simulink model "PubIfDecisionTOS_MDL"  (R2020b)
settings: configuration reference "DspaceConfig" (kept outside this file)
PostLoadFcn:
  | if any(exist('dsrtsu_mdlpostloadfcn', 'file') ~= 0), dsrtsu_mdlpostloadfcn('Execute', bdroot); end
InitFcn:
  | , if any(exist('dsmpb_private', 'file') ~= 0), dsmpb_private('dsmpb_mdlclblib', 'Init', bdroot); end,
undefined symbols (not defined in the file or in its folder): C_TOS_ACCEgoRAxletoFbumplength_m, C_TOS_ACCTargetFront_Flag, C_TOS_AEBJAPedObjDxThre_Val, C_TOS_AEBJAPedObjDyThre_Val, C_TOS_AEBJATargetSize_Val, C_TOS_AEBJAVehObjDxThre_Val, C_TOS_AEBJAVehObjDyThre_Val, C_TOS_AEBJuncPedTargetSize_Val, C_TOS_AEBLatObjDxThre_Val, C_TOS_AEBLatPedDyThre_Val, C_TOS_AEBLatTargetSize_Val, C_TOS_AEBLongTargetInEgoFront_Flag, C_TOS_axAbsGround_Parameter, C_TOS_CameraConfirmedFlag, C_TOS_CNsubjWidth, C_TOS_CurrentLaneCoreMinWidth_Val, C_TOS_CutInProb_Val_Zero, C_TOS_CutOutProb_Val_Zero, C_TOS_D2R_Val, C_TOS_DefaultValueObjectToCenterLine_dy, C_TOS_EgoCarWidth_Val, C_TOS_EgoDxRefPoint_m, C_TOS_EgoRAxletoFbumplength_m, C_TOS_HalfWidthVehicle_Con, C_TOS_HWA_CurrentLaneFlag, C_TOS_HWA_LeftLaneFlag, C_TOS_HWA_MovingDir_Vaild, C_TOS_HWA_MovState_Vaild, C_TOS_HWA_RightLaneFlag, C_TOS_LaneLineCourseErrorFront, C_TOS_LaneLineCourseErrorRear, C_TOS_MotorbikeDefaultWidth_m, C_TOS_NumberOfEffectiveTargets, C_TOS_Obj_Age_Val, C_TOS_Objdx_Constraint_Val, C_TOS_ObjectDefaultWidth_m, C_TOS_ObjInCurrentLane_Val, C_TOS_ObjInCurrentLaneValid, C_TOS_ObjInLeftLaneValid, C_TOS_ObjInRightLaneValid, C_TOS_ObjNotInCurrentLane_Val, C_TOS_ObjNotREElementType, C_TOS_ObjPredictDis_dy_ConstantVal_Zeros, C_TOS_ObjToCenterLine_ConstantVal_Zeros, C_TOS_OFMObjIDInvilad_Val, C_TOS_PIL_LatDisCons_Val_zero, C_TOS_PIL_ObjectCutInFlag_b, C_TOS_PIL_ObjectCutOutFlag_b, C_TOS_PIL_ObjLaneProb_al_Val, C_TOS_PP_ObjFusType_FC_Confirm_b, C_TOS_PP_ObjFusType_FC_FR_Confirm_b, C_TOS_PP_ObjFusType_FR_Confirm_b, C_TOS_RE_80BoolDefault_Val, C_TOS_RE_80Single181Default_Val, C_TOS_RE_80Single255Default_Val, C_TOS_RE_80Uint8Default_Val, C_TOS_RE_D2R, C_TOS_RE_D_180_Val, C_TOS_RE_InvalidObjectID_Val, C_TOS_RE_InvalidTargetChainDir_Val ... (+142)
libraries: simulink x1650, TOS_LIB x361, canfdmsglib x14
(part 22 of 69)

== system PubIfDecisionTOS_MDL/TOS_20201112/TOS_2012080320/TOS/LC_LCKie_ELK/TOS_HWA/CurrentLane/HWA_Object_PreConfirm ==
  PP_ObjFusType_FC_FR_Confirm : Inport
  PP_ObjFusType_FR_Confirm : Inport  Port=2
  PP_ObjFusType_FC_Confirm : Inport  Port=3
  Object_ID : Inport  Port=4
  Obj_MovingState : Inport  Port=5
  Obj_Dx : Inport  Port=6
  Object_ObstacleProb : Inport  Port=7
  Object_DY : Inport  Port=8
  Object_Type : Inport  Port=9
  TOS_TLJ_SameLaneConfirm_Flag : Inport  Port=10
  LM_LR_Line04_fCamValid : Inport  Port=11
  LM_LR_Line05_fCamValid : Inport  Port=12
  LM_LR_Line06_fCamValid : Inport  Port=13
  PIL_OverlapRatio : Inport  Port=14
  LM_LR_Line04_dDisStart : Inport  Port=15
  LM_LR_Line04_dDisEnd : Inport  Port=16
  LM_LR_Line05_dDisStart : Inport  Port=17
  LM_LR_Line05_dDisEnd : Inport  Port=18
  LM_LR_Line06_dDisStart : Inport  Port=19
  LM_LR_Line06_dDisEnd : Inport  Port=20
  TOS_HWA_CurrentFront_Target_2_ID_K1 : Inport  Port=21
  TOS_HWA_CurrentFront_Target_2_Dx_K1 : Inport  Port=22
  Bus Creator : BusCreator  Inputs=10
  Constant : Constant  Value=10  OutDataTypeStr=uint8
  Delay : Delay  InitialCondition=0
  Selector1 : Selector  InputPortWidth=11  IndexOptions=Index vector (port)  Indices=[1 3]  OutputSizes=1
  Selector2 : Selector  InputPortWidth=11  IndexOptions=Index vector (port)  Indices=[1 3]  OutputSizes=1
  TOS_HWA_CurrentLaneFront_TargPreConfirm : Subsystem
  Unit Delay : UnitDelay  SampleTime=-1  HasFrameUpgradeWarning=on
  Unit Delay1 : UnitDelay  InitialCondition=255  SampleTime=-1  HasFrameUpgradeWarning=on
  Unit Delay2 : UnitDelay  SampleTime=-1  HasFrameUpgradeWarning=on
  TOS_HWA_CLF_TargetPreConfirm : Outport
  wires:
  PP_ObjFusType_FR_Confirm/1 -> TOS_HWA_CurrentLaneFront_TargPreConfirm/2(PP_ObjFusType_FR_Confirm)
  PP_ObjFusType_FC_FR_Confirm/1 -> TOS_HWA_CurrentLaneFront_TargPreConfirm/1(PP_ObjFusType_FC_FR_Confirm)
  PP_ObjFusType_FC_Confirm/1 -> TOS_HWA_CurrentLaneFront_TargPreConfirm/3(PP_ObjFusType_FC_Confirm)
  Object_ID/1 -> TOS_HWA_CurrentLaneFront_TargPreConfirm/4(Object_ID)
  TOS_HWA_CurrentFront_Target_2_Dx_K1/1 -> Selector2/1
  TOS_HWA_CurrentFront_Target_2_ID_K1/1 -> Selector1/1
  Object_DY/1 -> TOS_HWA_CurrentLaneFront_TargPreConfirm/8(Object_DY)
  Object_ObstacleProb/1 -> TOS_HWA_CurrentLaneFront_TargPreConfirm/7(Object_ObstacleProb)
  Obj_Dx/1 -> TOS_HWA_CurrentLaneFront_TargPreConfirm/6(Obj_Dx)
  Obj_MovingState/1 -> TOS_HWA_CurrentLaneFront_TargPreConfirm/5(Obj_MovingState)
  Object_Type/1 -> TOS_HWA_CurrentLaneFront_TargPreConfirm/9(Object_ObjType)
  Bus Creator/1 -> TOS_HWA_CLF_TargetPreConfirm/1  "TOS_HWA_CLF_TargetPre_ObserVale"
  PIL_OverlapRatio/1 -> Delay/1, Unit Delay2/1, TOS_HWA_CurrentLaneFront_TargPreConfirm/16(PIL_OverlapRatio)
  TOS_TLJ_SameLaneConfirm_Flag/1 -> TOS_HWA_CurrentLaneFront_TargPreConfirm/10(TOS_TLJ_SameLaneConfirm_Flag)
  TOS_HWA_CurrentLaneFront_TargPreConfirm/1(TOS_HWA_TargetPre_Filt_Flag) -> Bus Creator/1  "TOS_HWA_CLF_TargetPre_Filt_Flag"
  TOS_HWA_CurrentLaneFront_TargPreConfirm/2(TOS_HWA_TargetPre_1_ConditionFlag_ObserVale) -> Bus Creator/2  "TOS_HWA_CLF_TargetPre_1_ConditionFlag_ObserVale"
  TOS_HWA_CurrentLaneFront_TargPreConfirm/3(TOS_HWA_TargetPre_FusionTypeFlag_ObserVale) -> Bus Creator/3  "TOS_HWA_CLF_TargetPre_FusionTypeFlag_ObserVale"
  TOS_HWA_CurrentLaneFront_TargPreConfirm/4(TOS_HWA_TargetPre_PassedbyTarget_Flag_ObserVale) -> Bus Creator/4  "TOS_HWA_CLF_TargetPre_PassedbyTarget_Flag_ObserVale"
  TOS_HWA_CurrentLaneFront_TargPreConfirm/5(TOS_HWA_TargetPre_FenceFlag_ObserVale) -> Bus Creator/5  "TOS_HWA_CLF_TargetPre_FenceFlag_ObserVale"
  TOS_HWA_CurrentLaneFront_TargPreConfirm/6(TOS_HWA_TargetPre_ObjType_ObserVale) -> Bus Creator/6  "TOS_HWA_CLF_TargetPre_ObjType_ObserVale"
  TOS_HWA_CurrentLaneFront_TargPreConfirm/7(TOS_HWA_TargetPre_OverlapThre_Val_ObserVale) -> Bus Creator/7  "TOS_HWA_CLF_TargetPre_OverlapThre_Val_ObserVale"
  TOS_HWA_CurrentLaneFront_TargPreConfirm/8(TOS_HWA_TargetPre_SameLane_Flag) -> Bus Creator/8  "TOS_HWA_CLF_TargetPre_SameLane_Flag"
  TOS_HWA_CurrentLaneFront_TargPreConfirm/9(TOS_HWA_TargetPre_2_OverlapThre_ObserVale) -> Bus Creator/9  "TOS_HWA_CLF_TargetPre_2_OverlapThre_ObserVale"
  TOS_HWA_CurrentLaneFront_TargPreConfirm/10(TOS_HWA_TargetPre_3_SameLane_Flag_ObserVale) -> Bus Creator/10  "TOS_HWA_CLF_TargetPre_3_SameLane_Flag_ObserVale"
  Unit Delay/1 -> TOS_HWA_CurrentLaneFront_TargPreConfirm/14(TOS_HWA_CurrentFront_Target_2_ID_K1)
  Unit Delay1/1 -> TOS_HWA_CurrentLaneFront_TargPreConfirm/15(TOS_HWA_Dx_K1)
  Unit Delay2/1 -> TOS_HWA_CurrentLaneFront_TargPreConfirm/17(PIL_OverlapRatio_K1)
  Delay/1 -> TOS_HWA_CurrentLaneFront_TargPreConfirm/18(PIL_OverlapRatio_K2)
  LM_LR_Line04_fCamValid/1 -> TOS_HWA_CurrentLaneFront_TargPreConfirm/11(LM_LR_Line04_fCamValid)
  LM_LR_Line05_fCamValid/1 -> TOS_HWA_CurrentLaneFront_TargPreConfirm/12(LM_LR_Line05_fCamValid)
  LM_LR_Line06_fCamValid/1 -> TOS_HWA_CurrentLaneFront_TargPreConfirm/13(LM_LR_Line06_fCamValid)
  LM_LR_Line06_dDisEnd/1 -> TOS_HWA_CurrentLaneFront_TargPreConfirm/24(LM_LR_Line06_dDisEnd)
  LM_LR_Line04_dDisStart/1 -> TOS_HWA_CurrentLaneFront_TargPreConfirm/19(LM_LR_Line04_dDisStart)
  LM_LR_Line04_dDisEnd/1 -> TOS_HWA_CurrentLaneFront_TargPreConfirm/20(LM_LR_Line04_dDisEnd)
  LM_LR_Line05_dDisStart/1 -> TOS_HWA_CurrentLaneFront_TargPreConfirm/21(LM_LR_Line05_dDisStart)
  LM_LR_Line05_dDisEnd/1 -> TOS_HWA_CurrentLaneFront_TargPreConfirm/22(LM_LR_Line05_dDisEnd)
  LM_LR_Line06_dDisStart/1 -> TOS_HWA_CurrentLaneFront_TargPreConfirm/23(LM_LR_Line06_dDisStart)
  Selector1/1 -> Unit Delay/1
  Selector2/1 -> Unit Delay1/1
  Constant/1 -> Selector1/2, Selector2/2

== system PubIfDecisionTOS_MDL/TOS_20201112/TOS_2012080320/TOS/LC_LCKie_ELK/TOS_HWA/LeftLane/HWA_Object_PreConfirm ==
  PP_ObjFusType_FC_FR_Confirm : Inport
  PP_ObjFusType_FR_Confirm : Inport  Port=2
  PP_ObjFusType_FC_Confirm : Inport  Port=3
  Object_ID : Inport  Port=4
  Obj_MovingState : Inport  Port=5
  Obj_Dx : Inport  Port=6
  Object_ObstacleProb : Inport  Port=7
  Object_DY : Inport  Port=8
  Object_Type : Inport  Port=9
  Bus Creator : BusCreator  Inputs=5
  HWA_Object_PreConfirm : Subsystem
  TOS_HWA_LLF_TargetPreConfirm : Outport
  wires:
  PP_ObjFusType_FR_Confirm/1 -> HWA_Object_PreConfirm/2(PP_ObjFusType_FR_Confirm)
  PP_ObjFusType_FC_FR_Confirm/1 -> HWA_Object_PreConfirm/1(PP_ObjFusType_FC_FR_Confirm)
  PP_ObjFusType_FC_Confirm/1 -> HWA_Object_PreConfirm/3(PP_ObjFusType_FC_Confirm)
  Object_ID/1 -> HWA_Object_PreConfirm/4(Object_ID)
  Object_DY/1 -> HWA_Object_PreConfirm/8(Object_DY)
  Object_ObstacleProb/1 -> HWA_Object_PreConfirm/7(Object_ObstacleProb)
  Obj_Dx/1 -> HWA_Object_PreConfirm/6(Obj_Dx)
  Obj_MovingState/1 -> HWA_Object_PreConfirm/5(Obj_MovingState)
  Object_Type/1 -> HWA_Object_PreConfirm/9(Object_ObjType)
  Bus Creator/1 -> TOS_HWA_LLF_TargetPreConfirm/1  "TOS_HWA_LLF_TargetPreConfirm"
  HWA_Object_PreConfirm/1(TOS_HWA_TargetPre_Confirm_Filt_Flag) -> Bus Creator/1  "TOS_HWA_LLF_TargetPre_Confirm_Filt_Flag"
  HWA_Object_PreConfirm/2(TOS_HWA_TargetPre_FusionTypeFlag_ObserVale) -> Bus Creator/2  "TOS_HWA_LLF_TargetPre_FusionTypeFlag_ObserVale"
  HWA_Object_PreConfirm/3(TOS_HWA_TargetPre_PassedbyTarget_ObserVale) -> Bus Creator/3  "TOS_HWA_LLF_TargetPre_PassedbyTarget_ObserVale"
  HWA_Object_PreConfirm/4(TOS_HWA_TargetPre_ObjType_ObserVale) -> Bus Creator/4  "TOS_HWA_LLF_TargetPre_ObjType_ObserVale"
  HWA_Object_PreConfirm/5(TOS_HWA_DyConfirm_ObserVale) -> Bus Creator/5  "TOS_HWA_LLF_DyConfirm_ObserVale"

== system PubIfDecisionTOS_MDL/TOS_20201112/TOS_2012080320/TOS/LC_LCKie_ELK/TOS_HWA/LeftLane/TOS_HWA_LeftLane ==
  TOSAAt_OFM_TIL_VIE : Inport
  HWA_LeftLane_ObjIndex : Inport  Port=2
  Bus Creator : BusCreator  Inputs=2
  Bus Creator1 : BusCreator  Inputs=5
  Bus Creator2 : BusCreator  Inputs=3
  Bus Selector : BusSelector  OutputSignals=TOS_AddAttributes.PP_ObjMovingDirSignalProcessing,OFM_SignalVerification.Object_VX,OFM_SignalVerification.Object_VY,OFM_SignalVerification.Object_Type,OFM_SignalVerification.Object_MovingState,TLJ_TargetInLaneValidityJudg.TOS_TLJ_LeftLaneConfirm_Flag,OFM_SignalVerification.Object_DX,OFM_SignalVerification.Object_DY,OFM_SignalVerification.Object_Fus_Type,OFM_SignalVerification.Object_HeadingAngle,TOS_AddAttributes.PP_ObjFusType_FC_FR_Confirm,TOS_AddAttributes.PP_ObjFusType_FR_Confirm,TOS_AddAttributes.PP_ObjFusType_FC_Confirm,VIE_SignalVerification.vxvRefMs
  Selector2 : Selector  InputPortWidth=4  IndexOptions=Index vector (dialog)  Indices=[1]  OutputSizes=1
  Selector3 : Selector  InputPortWidth=4  IndexOptions=Index vector (dialog)  Indices=[2]  OutputSizes=1
  Selector6 : Selector  InputPortWidth=4  IndexOptions=Index vector (dialog)  Indices=[3]  OutputSizes=1
  Selector7 : Selector  InputPortWidth=4  IndexOptions=Index vector (dialog)  Indices=[4]  OutputSizes=1
  TOS_HWA_LeftLane : Subsystem
  Terminator4 : Terminator
  HWA_LeftFront_Target_1 : Outport
  HWA_LeftFront_Target_2 : Outport  Port=2
  HWA_LeftRear_Target_3 : Outport  Port=3
  HWA_LeftRear_Target_4 : Outport  Port=4
  TargetInLeftLane_b : Outport  Port=5
  wires:
  TOS_HWA_LeftLane/11(TOS_HWA_LeftRear_DyConfirm_ObserVale) -> Bus Creator1/5  "TOS_HWA_LeftRear_DyConfirm_ObserVale"
  TOS_HWA_LeftLane/10(TOS_HWA_LeftRear_TargetMovingDir_ObserVale) -> Bus Creator1/4  "TOS_HWA_LeftRear_TargetMovingDir_ObserVale"
  TOS_HWA_LeftLane/9(TOS_HWA_InLeftLane_Rear_Flag_ObserVale) -> Bus Creator1/3  "TOS_HWA_InLeftLane_Rear_Flag_ObserVale"
  TOS_HWA_LeftLane/8(TOS_HWA_LeftRear_FusionType_ObserVale) -> Bus Creator1/2  "TOS_HWA_LeftRear_FusionType_ObserVale"
  TOS_HWA_LeftLane/7(TOS_HWA_LeftRear_MovState_ObserVale) -> Bus Creator1/1  "TOS_HWA_LeftRear_MovState_ObserVale"
  TOS_HWA_LeftLane/6(TOS_HWA_LeftFront_TargMovDir_ObserVale) -> Bus Creator2/3  "TOS_HWA_LeftFront_TargMovDir_ObserVale"
  TOS_HWA_LeftLane/5(TOS_HWA_InLeftLane_Front_Flag_ObserVale) -> Bus Creator2/2  "TOS_HWA_InLeftLane_Front_Flag_ObserVale"
  TOS_HWA_LeftLane/4(TOS_HWA_LeftFront_FusType_ObserVale) -> Bus Creator2/1  "TOS_HWA_LeftFront_FusType_ObserVale"
  Bus Selector/8 -> TOS_HWA_LeftLane/9(Object_DY)  "<Object_DY>"
  Bus Creator2/1 -> Bus Creator/1  "HWA_LeftLane_Front_ObserVale"
  Bus Creator1/1 -> Bus Creator/2  "HWA_LeftLane_Rear_ObserVale"
  TOS_HWA_LeftLane/3(TOS_HWA_LeftRear_TargConfirm_b) -> Selector7/1, Selector6/1
  Bus Selector/7 -> TOS_HWA_LeftLane/8(Object_DX)  "<Object_DX>"
  Bus Creator/1 -> Terminator4/1  "TOS_HWA_LeftLane_ObserVale"
  Bus Selector/14 -> TOS_HWA_LeftLane/15(VIE_EgoVelocity)  "<vxvRefMs>"
  Bus Selector/13 -> TOS_HWA_LeftLane/14(PP_ObjFusType_FC_Confirm)  "<PP_ObjFusType_FC_Confirm>"
  Bus Selector/12 -> TOS_HWA_LeftLane/13(PP_ObjFusType_FR_Confirm)  "<PP_ObjFusType_FR_Confirm>"
  Bus Selector/11 -> TOS_HWA_LeftLane/12(PP_ObjFusType_FC_FR_Confirm)  "<PP_ObjFusType_FC_FR_Confirm>"
  Selector2/1 -> HWA_LeftFront_Target_1/1
  Selector3/1 -> HWA_LeftFront_Target_2/1
  TOS_HWA_LeftLane/2(TOS_HWA_LeftFront_TargConfirm_b) -> Selector3/1, Selector2/1
  Selector7/1 -> HWA_LeftRear_Target_4/1
  Selector6/1 -> HWA_LeftRear_Target_3/1
  HWA_LeftLane_ObjIndex/1 -> TOS_HWA_LeftLane/1(HLeftLane_ObjIndex)
  TOSAAt_OFM_TIL_VIE/1 -> Bus Selector/1
  Bus Selector/1 -> TOS_HWA_LeftLane/2(PP_ObjMovingDirSignalProcessing)  "<PP_ObjMovingDirSignalProcessing>"
  Bus Selector/2 -> TOS_HWA_LeftLane/3(Object_VX)  "<Object_VX>"
  Bus Selector/3 -> TOS_HWA_LeftLane/4(Object_VY)  "<Object_VY>"
  Bus Selector/4 -> TOS_HWA_LeftLane/5(Object_Type)  "<Object_Type>"
  Bus Selector/5 -> TOS_HWA_LeftLane/6(Object_MovingState)  "<Object_MovingState>"
  Bus Selector/6 -> TOS_HWA_LeftLane/7(TOS_TLJ_LeftLaneConfirm_Flag)  "<TOS_TLJ_LeftLaneConfirm_Flag>"
  Bus Selector/9 -> TOS_HWA_LeftLane/10(Object_Fus_Type)  "<Object_Fus_Type>"
  TOS_HWA_LeftLane/1(TOS_HWA_TargetInLeftLane_b) -> TargetInLeftLane_b/1
  Bus Selector/10 -> TOS_HWA_LeftLane/11(Object_HeadingAngle)  "<Object_HeadingAngle>"

== system PubIfDecisionTOS_MDL/TOS_20201112/TOS_2012080320/TOS/LC_LCKie_ELK/TOS_HWA/RightLane/HWA_Object_PreConfirm ==
  PP_ObjFusType_FC_FR_Confirm : Inport
  PP_ObjFusType_FR_Confirm : Inport  Port=2
  PP_ObjFusType_FC_Confirm : Inport  Port=3
  Object_ID : Inport  Port=4
  Obj_MovingState : Inport  Port=5
  Obj_Dx : Inport  Port=6
  Object_ObstacleProb : Inport  Port=7
  Object_DY : Inport  Port=8
  Object_Type : Inport  Port=9
  Bus Creator : BusCreator  Inputs=5
  HWA_Object_PreConfirm : Subsystem
  TOS_HWA_RLF_TargetPreConfirm : Outport
  wires:
  PP_ObjFusType_FR_Confirm/1 -> HWA_Object_PreConfirm/2(PP_ObjFusType_FR_Confirm)
  PP_ObjFusType_FC_FR_Confirm/1 -> HWA_Object_PreConfirm/1(PP_ObjFusType_FC_FR_Confirm)
  PP_ObjFusType_FC_Confirm/1 -> HWA_Object_PreConfirm/3(PP_ObjFusType_FC_Confirm)
  Object_ID/1 -> HWA_Object_PreConfirm/4(Object_ID)
  Object_DY/1 -> HWA_Object_PreConfirm/8(Object_DY)
  Object_ObstacleProb/1 -> HWA_Object_PreConfirm/7(Object_ObstacleProb)
  Obj_Dx/1 -> HWA_Object_PreConfirm/6(Obj_Dx)
  Obj_MovingState/1 -> HWA_Object_PreConfirm/5(Obj_MovingState)
  Object_Type/1 -> HWA_Object_PreConfirm/9(Object_ObjType)
  Bus Creator/1 -> TOS_HWA_RLF_TargetPreConfirm/1  "TOS_HWA_RLF_TargetPreConfirm"
  HWA_Object_PreConfirm/1(TOS_HWA_TargetPre_Confirm_Filt_Flag) -> Bus Creator/1  "TOS_HWA_RLF_TargetPre_Confirm_Filt_Flag"
  HWA_Object_PreConfirm/2(TOS_HWA_TargetPre_FusionTypeFlag_ObserVale) -> Bus Creator/2  "TOS_HWA_RLF_TargetPre_FusionTypeFlag_ObserVale"
  HWA_Object_PreConfirm/3(TOS_HWA_TargetPre_PassedbyTarget_ObserVale) -> Bus Creator/3  "TOS_HWA_RLF_TargetPre_PassedbyTarget_ObserVale"
  HWA_Object_PreConfirm/4(TOS_HWA_TargetPre_ObjType_ObserVale) -> Bus Creator/4  "TOS_HWA_RLF_TargetPre_ObjType_ObserVale"
  HWA_Object_PreConfirm/5(TOS_HWA_DyConfirm_ObserVale) -> Bus Creator/5  "TOS_HWA_RLF_DyConfirm_ObserVale"

== system PubIfDecisionTOS_MDL/TOS_20201112/TOS_2012080320/TOS/LC_LCKie_ELK/TOS_HWA/RightLane/TOS_HWA_RightLane ==
  TOSAAt_OFM_TIL_VIE : Inport
  HWA_RightLane_ObjIndex : Inport  Port=2
  Bus Creator : BusCreator  Inputs=2
  Bus Creator1 : BusCreator  Inputs=5
  Bus Creator2 : BusCreator  Inputs=3
  Bus Selector : BusSelector  OutputSignals=TOS_AddAttributes.PP_ObjMovingDirSignalProcessing,OFM_SignalVerification.Object_VX,OFM_SignalVerification.Object_VY,OFM_SignalVerification.Object_Type,OFM_SignalVerification.Object_MovingState,TLJ_TargetInLaneValidityJudg.TOS_TLJ_RightLaneConfirm_Flag,OFM_SignalVerification.Object_DX,OFM_SignalVerification.Object_DY,OFM_SignalVerification.Object_Fus_Type,OFM_SignalVerification.Object_HeadingAngle,TOS_AddAttributes.PP_ObjFusType_FC_FR_Confirm,TOS_AddAttributes.PP_ObjFusType_FR_Confirm,TOS_AddAttributes.PP_ObjFusType_FC_Confirm,VIE_SignalVerification.vxvRefMs
  Selector2 : Selector  InputPortWidth=4  IndexOptions=Index vector (dialog)  Indices=[1]  OutputSizes=1
  Selector3 : Selector  InputPortWidth=4  IndexOptions=Index vector (dialog)  Indices=[2]  OutputSizes=1
  Selector6 : Selector  InputPortWidth=4  IndexOptions=Index vector (dialog)  Indices=[3]  OutputSizes=1
  Selector7 : Selector  InputPortWidth=4  IndexOptions=Index vector (dialog)  Indices=[4]  OutputSizes=1
  TOS_HWA_RightLane : Subsystem
  Terminator4 : Terminator
  HWA_RightFront_Target_1 : Outport
  HWA_RightFront_Target_2 : Outport  Port=2
  HWA_RightRear_Target_3 : Outport  Port=3
  HWA_RightRear_Target_4 : Outport  Port=4
  TargetInRightLane_b : Outport  Port=5
  wires:
  Bus Selector/10 -> TOS_HWA_RightLane/11(Object_HeadingAngle)  "<Object_HeadingAngle>"
  TOS_HWA_RightLane/1(TOS_HWA_TargetInRightLane_b) -> TargetInRightLane_b/1
  Bus Selector/9 -> TOS_HWA_RightLane/10(Object_Fus_Type)  "<Object_Fus_Type>"
  Bus Selector/6 -> TOS_HWA_RightLane/7(TOS_TLJ_RightLaneConfirm_Flag)  "<TOS_TLJ_RightLaneConfirm_Flag>"
  Bus Selector/5 -> TOS_HWA_RightLane/6(Object_MovingState)  "<Object_MovingState>"
  Bus Selector/4 -> TOS_HWA_RightLane/5(Object_Type)  "<Object_Type>"
  Bus Selector/3 -> TOS_HWA_RightLane/4(Object_VY)  "<Object_VY>"
  Bus Selector/2 -> TOS_HWA_RightLane/3(Object_VX)  "<Object_VX>"
  Bus Selector/1 -> TOS_HWA_RightLane/2(PP_ObjMovingDirSignalProcessing)  "<PP_ObjMovingDirSignalProcessing>"
  TOSAAt_OFM_TIL_VIE/1 -> Bus Selector/1
  HWA_RightLane_ObjIndex/1 -> TOS_HWA_RightLane/1(HWA_RightLane_ObjIndex)
  Selector6/1 -> HWA_RightRear_Target_3/1
  Selector7/1 -> HWA_RightRear_Target_4/1
  TOS_HWA_RightLane/2(TOS_HWA_RightFront_TargConfirm_b) -> Selector2/1, Selector3/1
  Selector3/1 -> HWA_RightFront_Target_2/1
  Selector2/1 -> HWA_RightFront_Target_1/1
  Bus Selector/11 -> TOS_HWA_RightLane/12(PP_ObjFusType_FC_FR_Confirm)  "<PP_ObjFusType_FC_FR_Confirm>"
  Bus Selector/12 -> TOS_HWA_RightLane/13(PP_ObjFusType_FR_Confirm)  "<PP_ObjFusType_FR_Confirm>"
  Bus Selector/13 -> TOS_HWA_RightLane/14(PP_ObjFusType_FC_Confirm)  "<PP_ObjFusType_FC_Confirm>"
  Bus Selector/14 -> TOS_HWA_RightLane/15(VIE_EgoVelocity)  "<vxvRefMs>"
  Bus Creator/1 -> Terminator4/1  "TOS_HWA_RightLane_ObserVale"
  Bus Selector/7 -> TOS_HWA_RightLane/8(Object_DX)  "<Object_DX>"
  TOS_HWA_RightLane/3(TOS_HWA_RightRear_TargConfirm_b) -> Selector6/1, Selector7/1
  Bus Creator1/1 -> Bus Creator/2  "HWA_RightLane_Rear_ObserVale"
  Bus Creator2/1 -> Bus Creator/1  "HWA_RightLane_Front_ObserVale"
  Bus Selector/8 -> TOS_HWA_RightLane/9(Object_DY)  "<Object_DY>"
  TOS_HWA_RightLane/4(TOS_HWA_RightFront_FusType_ObserVale) -> Bus Creator2/1  "TOS_HWA_RightFront_FusType_ObserVale"
  TOS_HWA_RightLane/5(TOS_HWA_InRightLane_Front_Flag_ObserVale) -> Bus Creator2/2  "TOS_HWA_InRightLane_Front_Flag_ObserVale"
  TOS_HWA_RightLane/6(TOS_HWA_RightFront_TargMovDir_ObserVale) -> Bus Creator2/3  "TOS_HWA_RightFront_TargMovDir_ObserVale"
  TOS_HWA_RightLane/7(TOS_HWA_RightRear_MovState_ObserVale) -> Bus Creator1/1  "TOS_HWA_RightRear_MovState_ObserVale"
  TOS_HWA_RightLane/8(TOS_HWA_RightRear_FusionType_ObserVale) -> Bus Creator1/2  "TOS_HWA_RightRear_FusionType_ObserVale"
  TOS_HWA_RightLane/9(TOS_HWA_InRightLane_Rear_Flag_ObserVale) -> Bus Creator1/3  "TOS_HWA_InRightLane_Rear_Flag_ObserVale"
  TOS_HWA_RightLane/10(TOS_HWA_RightRear_TargetMovingDir_ObserVale) -> Bus Creator1/4  "TOS_HWA_RightRear_TargetMovingDir_ObserVale"
  TOS_HWA_RightLane/11(TOS_HWA_RightRear_DyConfirm_ObserVale) -> Bus Creator1/5  "TOS_HWA_RightRear_DyConfirm_ObserVale"

== system PubIfDecisionTOS_MDL/TOS_20201112/TOS_2012080320/TOS/P0_Trajectory_V1.0/CordinatConvert/CordinatConvert/CordinatConvert ==
  EgoVeh_OffsetX : Inport
  EgoVeh_OffsetY : Inport  Port=2
  EgoVeh_OffsetAngle : Inport  Port=3
  P0_dx_TrackRecord_K1 : Inport  Port=4
  P0_dy_TrackRecord_K1 : Inport  Port=5
  P0_Counter_TrackRecord : Inport  Port=6
  P0_ID_TrackRecord_K1 : Inport  Port=7
  Action Port : ActionPort  ActionPortLabel=if(u1 == 1)
  TrackRecord_CordinatConvert : Subsystem  TreatAsAtomicUnit=on
  P0_dx_TrackRecord_CordinatConvert_K1 : Outport
  P0_dy_TrackRecord_CordinatConvert_K1 : Outport  Port=2
  P0_Counter_TrackRecord_CordinatConvert_K1 : Outport  Port=3
  P0_ID_TrackRecord_CordinatConvert_K1 : Outport  Port=4
  wires:
  TrackRecord_CordinatConvert/3(P0_Counter_TrackRecord_CordinatConvert_K1) -> P0_Counter_TrackRecord_CordinatConvert_K1/1
  P0_Counter_TrackRecord/1 -> TrackRecord_CordinatConvert/6(P0_Counter_TrackRecord)  "P0_Counter_TrackRecord"
  P0_dy_TrackRecord_K1/1 -> TrackRecord_CordinatConvert/5(P0_dy_TrackRecord_K1)  "P0_dy_TrackRecord_K1"
  P0_dx_TrackRecord_K1/1 -> TrackRecord_CordinatConvert/4(P0_dx_TrackRecord_K1)  "P0_dx_TrackRecord_K1"
  EgoVeh_OffsetAngle/1 -> TrackRecord_CordinatConvert/3(EgoVeh_OffsetAngle)  "EgoVeh_OffsetAngle"
  EgoVeh_OffsetY/1 -> TrackRecord_CordinatConvert/2(EgoVeh_OffsetY)  "EgoVeh_OffsetY"
  EgoVeh_OffsetX/1 -> TrackRecord_CordinatConvert/1(EgoVeh_OffsetX)  "EgoVeh_OffsetX"
  TrackRecord_CordinatConvert/2(P0_dy_TrackRecord_CordinatConvert_K1) -> P0_dy_TrackRecord_CordinatConvert_K1/1
  TrackRecord_CordinatConvert/1(P0_dx_TrackRecord_CordinatConvert_K1) -> P0_dx_TrackRecord_CordinatConvert_K1/1
  P0_ID_TrackRecord_K1/1 -> TrackRecord_CordinatConvert/7(P0_ID_TrackRecord_K1)  "P0_ID_TrackRecord_K1"
  TrackRecord_CordinatConvert/4(P0_ID_TrackRecord_CordinatConvert_K1) -> P0_ID_TrackRecord_CordinatConvert_K1/1

== system PubIfDecisionTOS_MDL/TOS_20201112/TOS_2012080320/TOS/P0_Trajectory_V1.0/CordinatConvert/CordinatConvert/CordinatConvertDefault ==
  Action Port : ActionPort  ActionPortLabel=else
  Constant : Constant  Value=single(zeros(P_TOS_P0_Trajectory_TrackRecord_Num,1))
  Constant1 : Constant  Value=single(zeros(P_TOS_P0_Trajectory_TrackRecord_Num,1))
  Constant2 : Constant  Value=uint32(zeros(P_TOS_P0_Trajectory_TrackRecord_Num,1))
  Constant3 : Constant  Value=uint8(zeros(P_TOS_P0_Trajectory_TrackRecord_Num,1))
  P0_dx_TrackRecord_CordinatConvert_K1 : Outport
  P0_dy_TrackRecord_CordinatConvert_K1 : Outport  Port=2
  P0_Counter_TrackRecord_CordinatConvert_K1 : Outport  Port=3
  P0_ID_TrackRecord_CordinatConvert_K1 : Outport  Port=4
  wires:
  Constant2/1 -> P0_Counter_TrackRecord_CordinatConvert_K1/1
  Constant1/1 -> P0_dy_TrackRecord_CordinatConvert_K1/1
  Constant/1 -> P0_dx_TrackRecord_CordinatConvert_K1/1
  Constant3/1 -> P0_ID_TrackRecord_CordinatConvert_K1/1

== system PubIfDecisionTOS_MDL/TOS_20201112/TOS_2012080320/TOS/P0_Trajectory_V1.0/CordinatConvert/CordinatConvert1/CordinatConvert ==
  EgoVeh_OffsetX : Inport
  EgoVeh_OffsetY : Inport  Port=2
  EgoVeh_OffsetAngle : Inport  Port=3
  P0_dx_TrackRecord_K1 : Inport  Port=4
  P0_dy_TrackRecord_K1 : Inport  Port=5
  P0_Counter_TrackRecord : Inport  Port=6
  P0_ID_TrackRecord_K1 : Inport  Port=7
  Action Port : ActionPort
  TrackRecord_CordinatConvert : Subsystem  TreatAsAtomicUnit=on
  P0_dx_TrackRecord_CordinatConvert_K1 : Outport
  P0_dy_TrackRecord_CordinatConvert_K1 : Outport  Port=2
  P0_Counter_TrackRecord_CordinatConvert_K1 : Outport  Port=3
  P0_ID_TrackRecord_CordinatConvert_K1 : Outport  Port=4
  wires:
  TrackRecord_CordinatConvert/4(P0_ID_TrackRecord_CordinatConvert_K1) -> P0_ID_TrackRecord_CordinatConvert_K1/1
  P0_ID_TrackRecord_K1/1 -> TrackRecord_CordinatConvert/7(P0_ID_TrackRecord_K1)  "P0_ID_TrackRecord_K1"
  TrackRecord_CordinatConvert/1(P0_dx_TrackRecord_CordinatConvert_K1) -> P0_dx_TrackRecord_CordinatConvert_K1/1
  TrackRecord_CordinatConvert/2(P0_dy_TrackRecord_CordinatConvert_K1) -> P0_dy_TrackRecord_CordinatConvert_K1/1
  EgoVeh_OffsetX/1 -> TrackRecord_CordinatConvert/1(EgoVeh_OffsetX)  "EgoVeh_OffsetX"
  EgoVeh_OffsetY/1 -> TrackRecord_CordinatConvert/2(EgoVeh_OffsetY)  "EgoVeh_OffsetY"
  EgoVeh_OffsetAngle/1 -> TrackRecord_CordinatConvert/3(EgoVeh_OffsetAngle)  "EgoVeh_OffsetAngle"
  P0_dx_TrackRecord_K1/1 -> TrackRecord_CordinatConvert/4(P0_dx_TrackRecord_K1)  "P0_dx_TrackRecord_K1"
  P0_dy_TrackRecord_K1/1 -> TrackRecord_CordinatConvert/5(P0_dy_TrackRecord_K1)  "P0_dy_TrackRecord_K1"
  P0_Counter_TrackRecord/1 -> TrackRecord_CordinatConvert/6(P0_Counter_TrackRecord)  "P0_Counter_TrackRecord"
  TrackRecord_CordinatConvert/3(P0_Counter_TrackRecord_CordinatConvert_K1) -> P0_Counter_TrackRecord_CordinatConvert_K1/1

== system PubIfDecisionTOS_MDL/TOS_20201112/TOS_2012080320/TOS/P0_Trajectory_V1.0/CordinatConvert/CordinatConvert1/CordinatConvertDefault ==
  Action Port : ActionPort
  Constant : Constant  Value=single(zeros(P0_Trajectory_TrackRecord_Num,1))
  Constant1 : Constant  Value=single(zeros(P0_Trajectory_TrackRecord_Num,1))
  Constant2 : Constant  Value=uint32(zeros(P0_Trajectory_TrackRecord_Num,1))
  Constant3 : Constant  Value=uint8(zeros(P0_Trajectory_TrackRecord_Num,1))
  P0_dx_TrackRecord_CordinatConvert_K1 : Outport
  P0_dy_TrackRecord_CordinatConvert_K1 : Outport  Port=2
  P0_Counter_TrackRecord_CordinatConvert_K1 : Outport  Port=3
  P0_ID_TrackRecord_CordinatConvert_K1 : Outport  Port=4
  wires:
  Constant3/1 -> P0_ID_TrackRecord_CordinatConvert_K1/1
  Constant/1 -> P0_dx_TrackRecord_CordinatConvert_K1/1
  Constant1/1 -> P0_dy_TrackRecord_CordinatConvert_K1/1
  Constant2/1 -> P0_Counter_TrackRecord_CordinatConvert_K1/1

== system PubIfDecisionTOS_MDL/TOS_20201112/TOS_2012080320/TOS/P0_Trajectory_V1.0/DataConfirm/Subsystem2/For Iterator Subsystem ==
  P0_dx_TrackRecord : Inport
  P0_dy_TrackRecord : Inport  Port=2
  P0_Counter_TrackRecord : Inport  Port=3
  P0_StartPosition_Num : Inport  Port=4
  P0_EndPosition_Num : Inport  Port=5
  Add : Sum  Inputs=++-
  Assignment1 : Assignment  DiagnosticForDimensions=Warning  IndexOptions=Index vector (port)  Indices=1  OutputSizes=1
  Assignment2 : Assignment  DiagnosticForDimensions=Warning  IndexOptions=Index vector (port)  Indices=1  OutputSizes=1
  Assignment4 : Assignment  DiagnosticForDimensions=Warning  IndexOptions=Index vector (port)  Indices=1  OutputSizes=1
  Constant : Constant  OutDataTypeStr=uint32
  Constant1 : Constant  Value=single(zeros(80,1))  OutDataTypeStr=uint32
      settings: AttributesFormatString=P0_Trajectory_TrackRecord_Num = unit32(60)
  Constant2 : Constant  Value=single(zeros(80,1))  OutDataTypeStr=single
      settings: AttributesFormatString=P0_Trajectory_TrackRecord_Num = unit32(60)
  For Iterator : ForIterator  IterationLimit=80
  Index Vector : MultiPortSwitch  Inputs=1
  Index Vector1 : MultiPortSwitch  Inputs=1
  Index Vector2 : MultiPortSwitch  Inputs=1
  Saturation : Saturate  UpperLimit=uint32(P_TOS_P0_Trajectory_TrackRecord_Num)  LowerLimit=uint32(1)
  Terminator : Terminator
  dx : Outport
  dy : Outport  Port=2
  P0_Counter : Outport  Port=3
  wires:
  Assignment1/1 -> dx/1
  Assignment4/1 -> P0_Counter/1
  Index Vector/1 -> Assignment1/2
  Assignment2/1 -> dy/1
  Constant2/1 -> Assignment2/1, Assignment1/1
  For Iterator/1 -> Assignment1/3, Assignment2/3, Assignment4/3, Add/2
  P0_dx_TrackRecord/1 -> Index Vector/2
  P0_StartPosition_Num/1 -> Add/1
  Add/1 -> Saturation/1
  Constant/1 -> Add/3
  P0_dy_TrackRecord/1 -> Index Vector1/2
  Index Vector1/1 -> Assignment2/2
  Index Vector2/1 -> Assignment4/2
  P0_Counter_TrackRecord/1 -> Index Vector2/2
  P0_EndPosition_Num/1 -> Terminator/1
  Saturation/1 -> Index Vector2/1, Index Vector1/1, Index Vector/1
  Constant1/1 -> Assignment4/1

== system PubIfDecisionTOS_MDL/TOS_20201112/TOS_2012080320/TOS/P0_Trajectory_V1.0/DataConfirm/Subsystem3/For Iterator Subsystem ==
  P0_dx_TrackRecord : Inport
  P0_dy_TrackRecord : Inport  Port=2
  P0_Counter_TrackRecord : Inport  Port=3
  P0_StartPosition_Num : Inport  Port=4
  P0_EndPosition_Num : Inport  Port=5
  Add : Sum  Inputs=++-
  Add1 : Sum  Inputs=++-
  Add2 : Sum  Inputs=+-
  Add3 : Sum  Inputs=++-
  Assignment1 : Assignment  DiagnosticForDimensions=Warning  IndexOptions=Index vector (port)  Indices=1  OutputSizes=1
  Assignment2 : Assignment  DiagnosticForDimensions=Warning  IndexOptions=Index vector (port)  Indices=1  OutputSizes=1
  Assignment3 : Assignment  DiagnosticForDimensions=Warning  IndexOptions=Index vector (port)  Indices=1  OutputSizes=1
  Constant : Constant  Value=80  OutDataTypeStr=int32
  Constant1 : Constant  OutDataTypeStr=int32
  Constant2 : Constant  Value=single(zeros(80,1))  OutDataTypeStr=single
      settings: AttributesFormatString=P0_Trajectory_TrackRecord_Num = unit32(60)
  Constant3 : Constant  OutDataTypeStr=uint32
  Constant4 : Constant  Value=single(zeros(80,1))  OutDataTypeStr=single
      settings: AttributesFormatString=P0_Trajectory_TrackRecord_Num = unit32(60)
  Constant5 : Constant  Value=80  OutDataTypeStr=int32
  Constant6 : Constant  Value=single(zeros(80,1))  OutDataTypeStr=uint32
      settings: AttributesFormatString=P0_Trajectory_TrackRecord_Num = unit32(60)
  Constant8 : Constant  OutDataTypeStr=int32
  For Iterator : ForIterator  IterationLimit=80
  Index Vector{,1..5} (6 alike) : MultiPortSwitch  Inputs=1
  P0_StartPosition_Num1 : InportShadow  Port=4
  P0_StartPosition_Num2 : InportShadow  Port=4
  Relational Operator : RelationalOperator  Operator=<=  OutDataTypeStr=boolean  RndMeth=Simplest
  Saturation : Saturate  UpperLimit=uint32(P_TOS_P0_Trajectory_TrackRecord_Num)  LowerLimit=uint32(1)
  Saturation1 : Saturate  UpperLimit=uint32(P_TOS_P0_Trajectory_TrackRecord_Num)  LowerLimit=uint32(1)
  Switch : Switch  Criteria=u2 > Threshold
  Switch1 : Switch  Criteria=u2 > Threshold
  Switch2 : Switch  Criteria=u2 > Threshold
  Terminator : Terminator
  dx : Outport
  dy : Outport  Port=2
  P0_Counter : Outport  Port=3
  wires:
  P0_StartPosition_Num/1 -> Add1/1
  Constant/1 -> Add/1
  Constant1/1 -> Add/2
  P0_StartPosition_Num1/1 -> Add/3
  Add/1 -> Relational Operator/2
  P0_StartPosition_Num2/1 -> Add3/3
  Index Vector/1 -> Switch/1
  Assignment1/1 -> dx/1
  Add1/1 -> Saturation/1
  Constant3/1 -> Add1/3
  Saturation/1 -> [control_Flag1], Index Vector/1
  Constant2/1 -> Assignment1/1
  Add3/1 -> Add2/2
  Constant5/1 -> Add3/1
  Constant8/1 -> Add3/2
  For Iterator/1 -> Relational Operator/1, [Iterator]
  Saturation1/1 -> [control_Flag2], Index Vector3/1
  Add2/1 -> Saturation1/1
  P0_dx_TrackRecord/1 -> Index Vector3/2, Index Vector/2
  Index Vector3/1 -> Switch/3
  Switch/1 -> Assignment1/2
  [Iterator] -> Add1/2
  [Iterator] -> Add2/1
  [Iterator] -> Assignment1/3
  Assignment3/1 -> P0_Counter/1
  P0_EndPosition_Num/1 -> Terminator/1
  Index Vector4/1 -> Switch1/3
  Index Vector2/1 -> Switch1/1
  [control_Flag1] -> Index Vector2/1
  [control_Flag2] -> Index Vector4/1
  P0_dy_TrackRecord/1 -> Index Vector4/2, Index Vector2/2
  [Iterator] -> Assignment2/3
  Switch1/1 -> Assignment2/2
  Constant4/1 -> Assignment2/1
  Assignment2/1 -> dy/1
  Constant6/1 -> Assignment3/1
  Switch2/1 -> Assignment3/2
  [Iterator] -> Assignment3/3
  P0_Counter_TrackRecord/1 -> Index Vector1/2, Index Vector5/2
  [control_Flag2] -> Index Vector5/1
  [control_Flag1] -> Index Vector1/1
  Relational Operator/1 -> Switch2/2, Switch1/2, Switch/2
  Index Vector1/1 -> Switch2/1
  Index Vector5/1 -> Switch2/3

== system PubIfDecisionTOS_MDL/TOS_20201112/TOS_2012080320/TOS/P0_Trajectory_V1.0/TrackRecord/Subsystem1/P0_Position_Num ==
  P0_dx_TrackRecord_CordinatConvert_K1 : Inport
  P0_dy_TrackRecord_CordinatConvert_K1 : Inport  Port=2
  P0_ObjVaild_TrackRecord_CordinatConvert_K1 : Inport  Port=3
  P0_Trajectory_TrackRecord_Num : Inport  Port=4
  EndPosition : Subsystem
  For Iterator : ForIterator  IterationSource=external
  StartPosition : Subsystem
  P0_StartPosition_Num : Outport
  P0_StartPosition_Dis : Outport  Port=2
  P0_EndPosition_Num : Outport  Port=3
  P0_EndPosition_dx : Outport  Port=4
  P0_EndPosition_dy : Outport  Port=5
  wires:
  P0_dx_TrackRecord_CordinatConvert_K1/1 -> EndPosition/1(P0_dx_TrackRecord_CordinatConvert_K1), StartPosition/1(P0_dx_TrackRecord_CordinatConvert_K1)
  P0_dy_TrackRecord_CordinatConvert_K1/1 -> StartPosition/2(P0_dy_TrackRecord_CordinatConvert_K1), EndPosition/2(P0_dy_TrackRecord_CordinatConvert_K1)
  P0_ObjVaild_TrackRecord_CordinatConvert_K1/1 -> StartPosition/3(P0_ObjVaild_TrackRecord_CordinatConvert_K1), EndPosition/3(P0_ObjVaild_TrackRecord_CordinatConvert_K1)
  P0_Trajectory_TrackRecord_Num/1 -> For Iterator/1
  StartPosition/1(P0_StartPosition_Num) -> P0_StartPosition_Num/1
  StartPosition/2(P0_StartPosition_Dis) -> P0_StartPosition_Dis/1
  EndPosition/1(P0_EndPosition_Num) -> P0_EndPosition_Num/1
  EndPosition/2(P0_EndPosition_dx) -> P0_EndPosition_dx/1
  EndPosition/3(P0_EndPosition_dy) -> P0_EndPosition_dy/1
  For Iterator/1 -> EndPosition/4(P0_Trajectory_TrackRecord_Num), StartPosition/4(P0_Trajectory_TrackRecord_Num)

== system PubIfDecisionTOS_MDL/TOS_20201112/TOS_2012080320/TOS/P0_Trajectory_V1.0/TrackRecord/Subsystem2/P0_Position_Num ==
  P0_dx_TrackRecord_CordinatConvert_K1 : Inport
  P0_dy_TrackRecord_CordinatConvert_K1 : Inport  Port=2
  P0_ObjVaild_TrackRecord_CordinatConvert_K1 : Inport  Port=3
  P0_Trajectory_TrackRecord_Num : Inport  Port=4
  Abs : Abs
  Abs1 : Abs
  Abs2 : Abs
  Add : Sum  OutDataTypeStr=int32
  Add1 : Sum
  Compare To Constant1 : simulink/Logic and Bit Operations/Compare To Constant  relop===  const=single(0)  OutDataTypeStr=boolean
      settings: AttributesFormatString=single(0)
  Compare To Constant10 : simulink/Logic and Bit Operations/Compare To Constant  relop=~=  const=uint32(0)  OutDataTypeStr=boolean
      settings: AttributesFormatString=uint32(0)
  Compare To Constant2 : simulink/Logic and Bit Operations/Compare To Constant  relop===  const=uint32(0)  OutDataTypeStr=boolean
      settings: AttributesFormatString=uint32(0)
  Compare To Constant5 : simulink/Logic and Bit Operations/Compare To Constant  relop===  const=single(0)  OutDataTypeStr=boolean
      settings: AttributesFormatString=single(0)
  Constant : Constant  OutDataTypeStr=int32
  Constant1 : Constant  OutDataTypeStr=uint32
  Data Type Conversion : DataTypeConversion  OutDataTypeStr=uint32
  For Iterator : ForIterator  IterationSource=external
  Index Vector{,1..4} (5 alike) : MultiPortSwitch  Inputs=1
  Logical Operator2 : Logic  Inputs=4  AllPortsSameDT=off  OutDataTypeStr=boolean
  P0_dx_TrackRecord_CordinatConvert_K2 : InportShadow
  Saturation : Saturate  UpperLimit=int32(P_TOS_P0_Trajectory_TrackRecord_Num)  LowerLimit=int32(1)
  Saturation1 : Saturate  UpperLimit=int32(P_TOS_P0_Trajectory_TrackRecord_Num)  LowerLimit=int32(1)
  Switch : Switch  Criteria=u2 > Threshold
  Unit Delay13 : UnitDelay  InitialCondition=uint32(1)  SampleTime=-1  HasFrameUpgradeWarning=on
      settings: AttributesFormatString=%<InitialCondition>
  P0_StartPosition_Num : Outport
  P0_StartPosition_Dis : Outport  Port=2
  wires:
  Index Vector1/1 -> Abs/1
  P0_dx_TrackRecord_CordinatConvert_K1/1 -> Index Vector1/2
  P0_Trajectory_TrackRecord_Num/1 -> For Iterator/1
  P0_dy_TrackRecord_CordinatConvert_K1/1 -> Index Vector/2
  P0_ObjVaild_TrackRecord_CordinatConvert_K1/1 -> Index Vector3/2, Index Vector2/2
  Index Vector2/1 -> Abs2/1
  Index Vector/1 -> Abs1/1
  Abs1/1 -> Compare To Constant5/1
  Abs/1 -> Compare To Constant1/1
  Abs2/1 -> Compare To Constant2/1
  Constant/1 -> Add/1
  Add/1 -> Saturation/1
  Saturation/1 -> Index Vector3/1
  Compare To Constant5/1 -> Logical Operator2/1
  Compare To Constant1/1 -> Logical Operator2/2
  Compare To Constant2/1 -> Logical Operator2/3
  Index Vector3/1 -> Compare To Constant10/1
  Compare To Constant10/1 -> Logical Operator2/4
  Add1/1 -> Saturation1/1
  Unit Delay13/1 -> Switch/3
  Data Type Conversion/1 -> Add1/2
  Constant1/1 -> Add1/1
  Saturation1/1 -> Switch/1
  For Iterator/1 -> Index Vector/1, Add/2, Index Vector2/1, Index Vector1/1, Data Type Conversion/1
  Index Vector4/1 -> P0_StartPosition_Dis/1
  Switch/1 -> Index Vector4/1, Unit Delay13/1, P0_StartPosition_Num/1
  P0_dx_TrackRecord_CordinatConvert_K2/1 -> Index Vector4/2
  Logical Operator2/1 -> Switch/2

== system PubIfDecisionTOS_MDL/TOS_20201112/TOS_2012080320/TOS/P0_Trajectory_V1.0/TrackRecord/Subsystem3/P0_Position_Num ==
  P0_dx_TrackRecord_CordinatConvert_K1 : Inport
  P0_dy_TrackRecord_CordinatConvert_K1 : Inport  Port=2
  P0_ObjVaild_TrackRecord_CordinatConvert_K1 : Inport  Port=3
  P0_Trajectory_TrackRecord_Num : Inport  Port=4
  Abs : Abs
  Abs1 : Abs
  Abs2 : Abs
  Add : Sum  OutDataTypeStr=int32
  Add1 : Sum
  Compare To Constant1 : simulink/Logic and Bit Operations/Compare To Constant  relop===  const=single(0)  OutDataTypeStr=boolean
      settings: AttributesFormatString=single(0)
  Compare To Constant10 : simulink/Logic and Bit Operations/Compare To Constant  relop=~=  const=uint32(0)  OutDataTypeStr=boolean
      settings: AttributesFormatString=uint32(0)
  Compare To Constant2 : simulink/Logic and Bit Operations/Compare To Constant  relop===  const=uint32(0)  OutDataTypeStr=boolean
      settings: AttributesFormatString=uint32(0)
  Compare To Constant5 : simulink/Logic and Bit Operations/Compare To Constant  relop===  const=single(0)  OutDataTypeStr=boolean
      settings: AttributesFormatString=single(0)
  Constant : Constant  OutDataTypeStr=int32
  Constant1 : Constant  OutDataTypeStr=uint32
  Data Type Conversion : DataTypeConversion  OutDataTypeStr=uint32
  For Iterator : ForIterator  IterationSource=external
  Index Vector{,1..4} (5 alike) : MultiPortSwitch  Inputs=1
  Logical Operator2 : Logic  Inputs=4  AllPortsSameDT=off  OutDataTypeStr=boolean
  P0_dx_TrackRecord_CordinatConvert_K2 : InportShadow
  Saturation : Saturate  UpperLimit=int32(P_TOS_P0_Trajectory_TrackRecord_Num)  LowerLimit=int32(1)
  Saturation1 : Saturate  UpperLimit=int32(P_TOS_P0_Trajectory_TrackRecord_Num)  LowerLimit=int32(1)
  Switch : Switch  Criteria=u2 > Threshold
  Unit Delay13 : UnitDelay  InitialCondition=uint32(1)  SampleTime=-1  HasFrameUpgradeWarning=on
      settings: AttributesFormatString=%<InitialCondition>
  P0_StartPosition_Num : Outport
  P0_StartPosition_Dis : Outport  Port=2
  wires:
  Index Vector1/1 -> Abs/1
  P0_dx_TrackRecord_CordinatConvert_K1/1 -> Index Vector1/2
  P0_Trajectory_TrackRecord_Num/1 -> For Iterator/1
  P0_dy_TrackRecord_CordinatConvert_K1/1 -> Index Vector/2
  P0_ObjVaild_TrackRecord_CordinatConvert_K1/1 -> Index Vector3/2, Index Vector2/2
  Index Vector2/1 -> Abs2/1
  Index Vector/1 -> Abs1/1
  Abs1/1 -> Compare To Constant5/1
  Abs/1 -> Compare To Constant1/1
  Abs2/1 -> Compare To Constant2/1
  Constant/1 -> Add/1
  Add/1 -> Saturation/1
  Saturation/1 -> Index Vector3/1
  Compare To Constant5/1 -> Logical Operator2/1
  Compare To Constant1/1 -> Logical Operator2/2
  Compare To Constant2/1 -> Logical Operator2/3
  Index Vector3/1 -> Compare To Constant10/1
  Compare To Constant10/1 -> Logical Operator2/4
  Logical Operator2/1 -> Switch/2
  Add1/1 -> Saturation1/1
  For Iterator/1 -> Index Vector/1, Add/2, Index Vector2/1, Index Vector1/1, Data Type Conversion/1
  Unit Delay13/1 -> Switch/3
  Switch/1 -> P0_StartPosition_Num/1, Index Vector4/1, Unit Delay13/1
  Data Type Conversion/1 -> Add1/2
  Constant1/1 -> Add1/1
  Saturation1/1 -> Switch/1
  P0_dx_TrackRecord_CordinatConvert_K2/1 -> Index Vector4/2
  Index Vector4/1 -> P0_StartPosition_Dis/1

== system PubIfDecisionTOS_MDL/TOS_20201112/TOS_2012080320/TOS/P0_Trajectory_V1.0/TrgValidConfirm/TrgValidConfirm/TrgValidConfirm ==
  note: 1.有效目标ID跳变处理
  dxP0 : Inport
  ObjDYP0 : Inport  Port=2
  IDP0 : Inport  Port=3
  P0_ID_K1 : Inport  Port=4
  P0_Counter_K1 : Inport  Port=5
  P0_dx_K1 : Inport  Port=6
  Action Port : ActionPort  ActionPortLabel=else
  Bus Creator : BusCreator  Inputs=6
  Bus Selector : BusSelector  OutputSignals=IDP0
  Compare To Constant : simulink/Logic and Bit Operations/Compare To Constant  relop=~=  const=C_TOS_OFMObjIDInvilad_Val  OutDataTypeStr=boolean
      settings: AttributesFormatString=C_TOS_OFMObjIDInvilad_Val = 0
  If : If  IfExpression=u1 == 1
  Merge{1..4} (4 alike) : Merge
  TrgValidConfirm : Subsystem  TreatAsAtomicUnit=on
  TrgValidConfirm_Default : Subsystem  TreatAsAtomicUnit=on
  P0_ID : Outport
  P0_Counter : Outport  Port=2
  P0_dx : Outport  Port=3
  P0_dy : Outport  Port=4
  wires:
  TrgValidConfirm/4(P0_dy) -> Merge4/1
  TrgValidConfirm/3(P0_dx) -> Merge3/1
  TrgValidConfirm/1(P0_ID) -> Merge1/1
  TrgValidConfirm/2(P0_Counter) -> Merge2/1
  TrgValidConfirm_Default/4(P0_dy) -> Merge4/2
  TrgValidConfirm_Default/3(P0_dx) -> Merge3/2
  TrgValidConfirm_Default/1(P0_ID) -> Merge1/2
  Compare To Constant/1 -> If/1
  P0_dx_K1/1 -> Bus Creator/6  "P0_dx_K1"
  Merge4/1 -> P0_dy/1
  Merge3/1 -> P0_dx/1
  Merge1/1 -> P0_ID/1
  Bus Creator/1 -> Bus Selector/1, [TrgValidConfirm_inf]
  P0_Counter_K1/1 -> Bus Creator/5  "P0_Counter_K1"
  P0_ID_K1/1 -> Bus Creator/4  "P0_ID_K1"
  IDP0/1 -> Bus Creator/3  "IDP0"
  ObjDYP0/1 -> Bus Creator/2  "ObjDYP0"
  dxP0/1 -> Bus Creator/1  "dxP0"
  Merge2/1 -> P0_Counter/1
  TrgValidConfirm_Default/2(P0_Counter) -> Merge2/2
  [TrgValidConfirm_inf] -> TrgValidConfirm/1(TrgValidConfirm_inf)
  If/2 -> TrgValidConfirm_Default/Action
  If/1 -> TrgValidConfirm/Action
  Bus Selector/1 -> Compare To Constant/1  "<IDP0>"

== system PubIfDecisionTOS_MDL/TOS_20201112/TOS_2012080320/TOS/P0_Trajectory_V1.0/TrgValidConfirm/TrgValidConfirm/TrgValidConfirmDefault ==
  Action Port : ActionPort  ActionPortLabel=if(u1 == 0)
  Constant1 : Constant  Value=0  OutDataTypeStr=single
  Constant2 : Constant  Value=0  OutDataTypeStr=uint32
  Constant3 : Constant  Value=0  OutDataTypeStr=single
  Constant4 : Constant  Value=0  OutDataTypeStr=uint8
  P0_ID : Outport
  P0_Counter : Outport  Port=2
  P0_dx : Outport  Port=3
  P0_dy : Outport  Port=4
  wires:
  Constant4/1 -> P0_ID/1
  Constant3/1 -> P0_dy/1
  Constant2/1 -> P0_Counter/1
  Constant1/1 -> P0_dx/1

== system PubIfDecisionTOS_MDL/TOS_20201112/TOS_2012080320/PIL_1029/BoundaryCalculat/Lane_BoundaryCalculat/Lane_Boundary/Boundary/LeftLane_BasicLaneWidth ==
  ObjectType : Inport
  object_MovingState : Inport  Port=2
  PP_LeftLaneWidth : Inport  Port=3
  Compare To Constant1 : simulink/Logic and Bit Operations/Compare To Constant  relop===  const=OFM_OBJ_TYPE_E.CAR  OutDataTypeStr=boolean
      settings: AttributesFormatString=OFM_OBJ_TYPE_E.CAR = 2
  Compare To Constant10 : simulink/Logic and Bit Operations/Compare To Constant  relop===  const=OFM_OBJ_MOVINGSTATE_E.UNKNOWN  OutDataTypeStr=boolean
      settings: AttributesFormatString=OFM_OBJ_MOVINGSTATE_E.UNKNOWN = 1
  Compare To Constant2 : simulink/Logic and Bit Operations/Compare To Constant  relop===  const=OFM_OBJ_TYPE_E.TRUCK  OutDataTypeStr=boolean
      settings: AttributesFormatString=OFM_OBJ_TYPE_E.TRUCK = 3
  Compare To Constant3 : simulink/Logic and Bit Operations/Compare To Constant  relop===  const=OFM_OBJ_TYPE_E.MOTORBIKE  OutDataTypeStr=boolean
      settings: AttributesFormatString=OFM_OBJ_TYPE_E.MOTORBIKE = 4
  Compare To Constant4 : simulink/Logic and Bit Operations/Compare To Constant  relop===  const=OFM_OBJ_TYPE_E.PEDESTRIAN  OutDataTypeStr=boolean
      settings: AttributesFormatString=OFM_OBJ_TYPE_E.PEDESTRIAN = 6
  Compare To Constant5 : simulink/Logic and Bit Operations/Compare To Constant  relop===  const=OFM_OBJ_TYPE_E.BICYCLE  OutDataTypeStr=boolean
      settings: AttributesFormatString=OFM_OBJ_TYPE_E.BICYCLE = 5
  Compare To Constant6 : simulink/Logic and Bit Operations/Compare To Constant  relop===  const=OFM_OBJ_TYPE_E.UNKNOWN_TYPE  OutDataTypeStr=boolean
      settings: AttributesFormatString=OFM_OBJ_TYPE_E.UNKNOWN_TYPE = 1
  Compare To Constant7 : simulink/Logic and Bit Operations/Compare To Constant  relop===  const=OFM_OBJ_TYPE_E.GENERAL_OBJECT  OutDataTypeStr=boolean
      settings: AttributesFormatString=OFM_OBJ_TYPE_E.GENERAL_OBJECT = 7
  Compare To Constant8 : simulink/Logic and Bit Operations/Compare To Constant  relop===  const=OFM_OBJ_TYPE_E.ANIMAL  OutDataTypeStr=boolean
      settings: AttributesFormatString=OFM_OBJ_TYPE_E.ANIMAL = 8
  Compare To Constant9 : simulink/Logic and Bit Operations/Compare To Constant  relop===  const=OFM_OBJ_MOVINGSTATE_E.STATIONARY  OutDataTypeStr=boolean
      settings: AttributesFormatString=OFM_OBJ_MOVINGSTATE_E.STATIONARY = 3
  Constant1 : Constant  Value=P_TOS_BasicLaneWidth_CAR_MinVal  OutDataTypeStr=single
      settings: AttributesFormatString=P_TOS_BasicLaneWidth_CAR_MinVal = 2.5
  Constant2 : Constant  Value=P_TOS_BasicLaneWidth_Pedestrian_MinVal  OutDataTypeStr=single
      settings: AttributesFormatString=P_TOS_BasicLaneWidth_Pedestrian_MinVal = 2
  Constant3 : Constant  Value=P_TOS_BasicLaneWidth_Bicycle_MinVal  OutDataTypeStr=single
      settings: AttributesFormatString=P_TOS_BasicLaneWidth_Bicycle_MinVal = 2.2
  Constant4 : Constant  Value=P_TOS_BasicLaneWidth_OthertType_MinVal  OutDataTypeStr=single
      settings: AttributesFormatString=P_TOS_BasicLaneWidth_OthertType_MinVal = 2.0
  Constant5 : Constant  Value=P_TOS_BasicLaneWidth_OthertType_MinVal  OutDataTypeStr=single
      settings: AttributesFormatString=P_TOS_BasicLaneWidth_OthertType_MinVal = 2.0
  Constant6 : Constant  Value=P_TOS_BasicLaneWidth_StillObj_MinVal  OutDataTypeStr=single
      settings: AttributesFormatString=P_TOS_BasicLaneWidth_StillObj_MinVal = 1.9
  Data Type Conversion : DataTypeConversion  OutDataTypeStr=Enum: OFM_OBJ_TYPE_E
  Data Type Conversion1 : DataTypeConversion  OutDataTypeStr=Enum: OFM_OBJ_MOVINGSTATE_E
  Logical Operator1 : Logic  Operator=OR  Inputs=3  AllPortsSameDT=off  OutDataTypeStr=boolean
  Logical Operator2 : Logic  Operator=OR  Inputs=3  AllPortsSameDT=off  OutDataTypeStr=boolean
  Logical Operator3 : Logic  Operator=OR  AllPortsSameDT=off  OutDataTypeStr=boolean
  MinMax : MinMax  Inputs=2  OutDataTypeStr=single
  Switch{1..5} (5 alike) : Switch  Criteria=u2 > Threshold
  LeftLane_BasicLaneWidth : Outport
  wires:
  Switch5/1 -> MinMax/2
  Constant6/1 -> Switch5/1
  Logical Operator3/1 -> Switch5/2
  Compare To Constant9/1 -> Logical Operator3/1
  Compare To Constant10/1 -> Logical Operator3/2
  MinMax/1 -> LeftLane_BasicLaneWidth/1
  PP_LeftLaneWidth/1 -> MinMax/1
  Compare To Constant2/1 -> Logical Operator1/2
  Data Type Conversion1/1 -> Compare To Constant10/1, Compare To Constant9/1
  Logical Operator1/1 -> Switch1/2
  Compare To Constant8/1 -> Logical Operator2/3
  Compare To Constant6/1 -> Logical Operator2/1
  Logical Operator2/1 -> Switch4/2
  Compare To Constant7/1 -> Logical Operator2/2
  Compare To Constant1/1 -> Logical Operator1/1
  Switch1/1 -> Switch5/3
  Compare To Constant3/1 -> Logical Operator1/3
  Switch3/1 -> Switch2/3
  Switch4/1 -> Switch3/3
  Switch2/1 -> Switch1/3
  Constant2/1 -> Switch2/1
  Constant4/1 -> Switch4/1
  Data Type Conversion/1 -> Compare To Constant3/1, Compare To Constant4/1, Compare To Constant5/1, Compare To Constant7/1, Compare To Constant8/1, Compare To Constant6/1, Compare To Constant2/1, Compare To Constant1/1
  Constant5/1 -> Switch4/3
  Compare To Constant5/1 -> Switch3/2
  Constant3/1 -> Switch3/1
  Constant1/1 -> Switch1/1
  Compare To Constant4/1 -> Switch2/2
  object_MovingState/1 -> Data Type Conversion1/1
  ObjectType/1 -> Data Type Conversion/1
